simulink model "untitled"  (R2023b)
settings: Solver=FixedStepDiscrete  StartTime=0.0  StopTime=10.0  FixedStep=Ts  RelTol=1e-3
values from neighbouring files (symbols this model uses):
  Ts = 0.01    [para.m]
settings Model: Creator=User  LastModifiedBy=User
settings OptimizationCC: DefaultParameterBehavior=Inlined  EnhancedBackFolding=on  PassReuseOutputArgsAs=Individual arguments  ZeroExternalMemoryAtStartup=off  ZeroInternalMemoryAtStartup=off  OptimizeBlockOrder=speed  DifferentSizesBufferReuse=on  OptimizationCustomize=off  EfficientTunableParamExpr=on
settings DebuggingCC: ParameterTunabilityLossMsg=error
settings HardwareCC: ProdBitPerPointer=32  ProdBitPerSizeT=32  ProdBitPerPtrDiffT=32  ProdLargestAtomicFloat=None  ProdWordSize=32  ProdHWDeviceType=Infineon->TriCore
settings SFSimCC: MATLABDynamicMemAlloc=off
settings RTWCC: Description=Embedded Coder  SystemTargetFile=ert.tlc  GenCodeOnly=on  TemplateMakefile=ert_default_tmf
settings CodeAppCC: ForceParamTrailComments=on  IgnoreCustomStorageClasses=off  OperatorAnnotations=on  SimulinkDataObjDesc=on  SFDataObjDesc=on  InsertBlockDesc=on
settings ERTTargetCC: TargetLangStandard=C99 (ISO)  GenerateSampleERTMain=on  InlinedParameterPlacement=NonHierarchical  ERTCustomFileTemplate=example_file_process.tlc

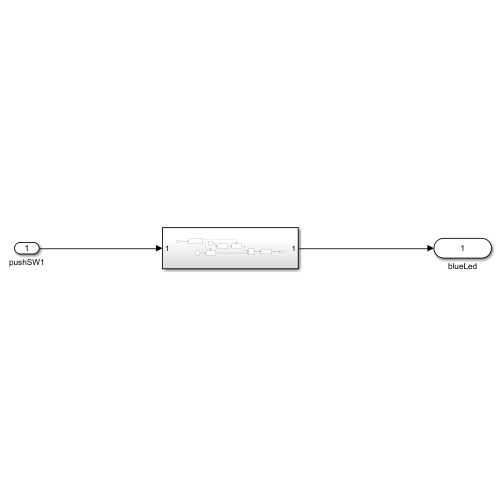
[thumbnail: Simulink's stored preview of the top-level diagram]
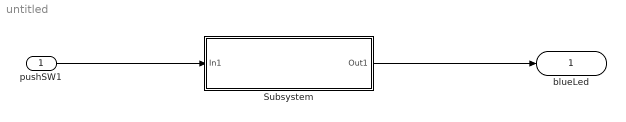
== system untitled ==
  pushSW1 : Inport  OutDataTypeStr=boolean
  Subsystem : Subsystem
  blueLed : Outport  OutDataTypeStr=uint16
  wires:
  pushSW1/1 -> Subsystem/1(In1)
  Subsystem/1(Out1) -> blueLed/1

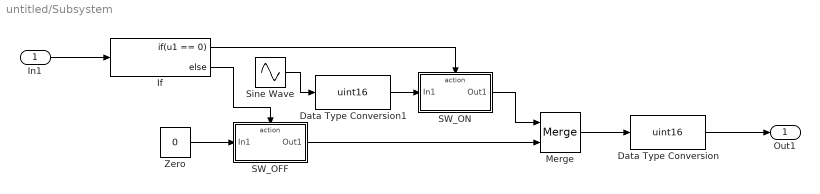
== system untitled/Subsystem ==
  In1 : Inport
  Data Type Conversion : DataTypeConversion  OutDataTypeStr=uint16  SaturateOnIntegerOverflow=off  RndMeth=Floor
  Data Type Conversion1 : DataTypeConversion  OutDataTypeStr=uint16  SaturateOnIntegerOverflow=off  RndMeth=Floor
  If : If  IfExpression=u1 == 0
  Merge : Merge
  SW_OFF : Subsystem  TreatAsAtomicUnit=on
  SW_ON : Subsystem  TreatAsAtomicUnit=on
  Sine Wave : Sin  SineType=Sample based  Amplitude=25000  Bias=25000  Frequency=300  Samples=300  SampleTime=Ts
  Zero : Constant  Value=0  OutDataTypeStr=uint16
  Out1 : Outport
  wires:
  SW_OFF/1(Out1) -> Merge/2
  Sine Wave/1 -> Data Type Conversion1/1
  If/2 -> SW_OFF/Action
  Zero/1 -> SW_OFF/1(In1)
  SW_ON/1(Out1) -> Merge/1
  Merge/1 -> Data Type Conversion/1
  Data Type Conversion1/1 -> SW_ON/1(In1)
  If/1 -> SW_ON/Action
  In1/1 -> If/1
  Data Type Conversion/1 -> Out1/1

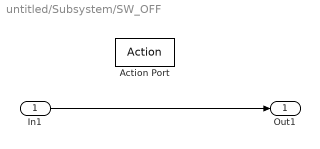
== system untitled/Subsystem/SW_OFF ==
  In1 : Inport
  Action Port : ActionPort  ActionPortLabel=else
  Out1 : Outport
  wires:
  In1/1 -> Out1/1

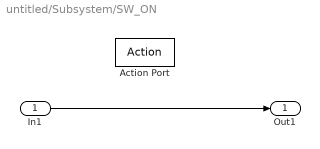
== system untitled/Subsystem/SW_ON ==
  In1 : Inport
  Action Port : ActionPort  ActionPortLabel=if(u1 == 0)
  Out1 : Outport
  wires:
  In1/1 -> Out1/1
